simulink model "MIMO_FLOATING_POINT"  (R2023b)
settings: Solver=VariableStepAuto  StartTime=0.0  StopTime=1000  RelTol=1e-3
libraries: dspsigops x80, commchan3 x4, commdigbbndpm3 x2, commfilt2 x2, commsink2 x1, simulink x1, commrandsrc3 x1
(part 2 of 3)

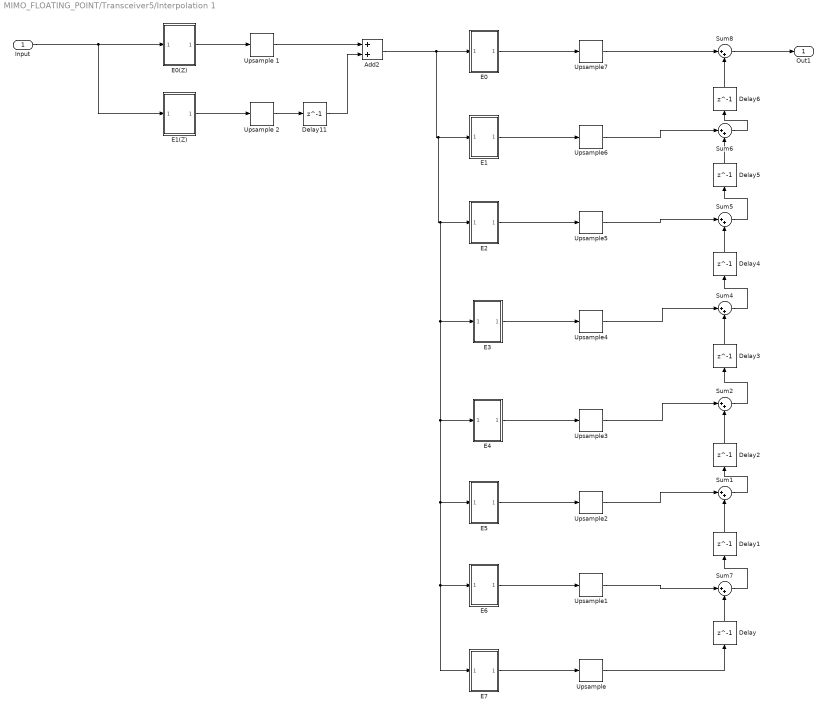
== system MIMO_FLOATING_POINT/Transceiver5/Interpolation 1 ==
  Input : Inport
  Add2 : Sum
  Delay{,1..6,11} (8 alike) : Delay  DelayLength=1
  E0 : Subsystem
  E0(Z) : Subsystem
  E1 : Subsystem
  E1(Z) : Subsystem
  E2 : Subsystem
  E3 : Subsystem
  E4 : Subsystem
  E5 : Subsystem
  E6 : Subsystem
  E7 : Subsystem
  Sum{1..2,4..8} (7 alike) : Sum  Inputs=|++
  Upsample{,1..7} (8 alike) : dspsigops/Upsample  N=8  phase=0  RateOptions=Allow multirate processing  ic=0  mode=Unused parameter value
  Upsample 1 : dspsigops/Upsample  N=2  phase=0  RateOptions=Allow multirate processing  ic=0  mode=Unused parameter value
  Upsample 2 : dspsigops/Upsample  N=2  phase=0  RateOptions=Allow multirate processing  ic=0  mode=Unused parameter value
  Out1 : Outport
  wires:
  Upsample/1 -> Delay/1
  Delay5/1 -> Sum6/2
  Add2/1 -> E7/1(In1), E6/1(In1), E5/1(In1), E4/1(In1), E3/1(In1), E2/1(In1), E1/1(In1), E0/1(In1)
  Upsample6/1 -> Sum6/1
  Delay4/1 -> Sum5/2
  Delay3/1 -> Sum4/2
  E5/1(Out1) -> Upsample2/1
  Sum6/1 -> Delay6/1
  Sum7/1 -> Delay1/1
  E7/1(Out1) -> Upsample/1
  Upsample1/1 -> Sum7/1
  Upsample2/1 -> Sum1/1
  Input/1 -> E1(Z)/1(Input1), E0(Z)/1(Input)
  E0(Z)/1(Out1) -> Upsample 1/1
  Upsample 2/1 -> Delay11/1
  Delay6/1 -> Sum8/2
  E0/1(Out1) -> Upsample7/1
  Delay/1 -> Sum7/2
  E1/1(Out1) -> Upsample6/1
  Delay1/1 -> Sum1/2
  Sum5/1 -> Delay5/1
  Sum4/1 -> Delay4/1
  Upsample5/1 -> Sum5/1
  Upsample 1/1 -> Add2/1
  Sum8/1 -> Out1/1
  Upsample4/1 -> Sum4/1
  Delay11/1 -> Add2/2
  Sum1/1 -> Delay2/1
  Sum2/1 -> Delay3/1
  E6/1(Out1) -> Upsample1/1
  E3/1(Out1) -> Upsample4/1
  Delay2/1 -> Sum2/2
  Upsample7/1 -> Sum8/1
  E1(Z)/1(Output) -> Upsample 2/1
  Upsample3/1 -> Sum2/1
  E2/1(Out1) -> Upsample5/1
  E4/1(Out1) -> Upsample3/1

== system MIMO_FLOATING_POINT/Transceiver5/Subsystem ==
  In1 : Inport
  Delay{,1,4..9} (8 alike) : Delay  DelayLength=1
  Delay2 : Delay  DelayLength=5
  Delay3 : Delay  DelayLength=3
  Gain : Gain
  Gain1 : Gain
  Gain2 : Gain
  Quantizer : Quantizer  QuantizationInterval=1
  Quantizer1 : Quantizer  QuantizationInterval=1
  Quantizer2 : Quantizer  QuantizationInterval=1
  Subtract : Sum  Inputs=+-
  Subtract1 : Sum  Inputs=+-
  Subtract2 : Sum  Inputs=+-
  Sum{,1..2,4,6} (5 alike) : Sum  Inputs=|++
  Sum3 : Sum  Inputs=|+-
  Sum5 : Sum  Inputs=|+-
  Out1 : Outport
  wires:
  Delay/1 -> Sum1/1, Gain/1
  Quantizer/1 -> Subtract/2, Delay2/1
  Sum/1 -> Subtract/1, Quantizer/1
  Sum2/1 -> Subtract2/1, Quantizer2/1
  Delay4/1 -> Gain2/1
  Delay8/1 -> Sum5/2
  Sum4/1 -> Sum5/1, Delay8/1
  Subtract/1 -> Delay/1
  Delay5/1 -> Delay6/1, Sum3/1
  Quantizer1/1 -> Subtract1/2, Delay3/1
  Delay1/1 -> Sum2/1, Gain1/1
  Gain2/1 -> Sum2/2
  Sum1/1 -> Subtract1/1, Quantizer1/1
  Subtract1/1 -> Delay1/1
  Gain1/1 -> Sum1/2
  Sum3/1 -> Delay7/1
  Gain/1 -> Sum/2
  Delay3/1 -> Sum4/1
  Delay7/1 -> Sum4/2
  Subtract2/1 -> Delay4/1
  Quantizer2/1 -> Subtract2/2, Delay5/1
  Delay6/1 -> Sum3/2
  Sum5/1 -> Delay9/1
  Delay2/1 -> Sum6/1
  Delay9/1 -> Sum6/2
  In1/1 -> Sum/1
  Sum6/1 -> Out1/1

== system MIMO_FLOATING_POINT/Transceiver5/Subsystem1 ==
  In1 : Inport
  Delay{,1,4..9} (8 alike) : Delay  DelayLength=1
  Delay2 : Delay  DelayLength=5
  Delay3 : Delay  DelayLength=3
  Gain : Gain
  Gain1 : Gain
  Gain2 : Gain
  Quantizer : Quantizer  QuantizationInterval=1
  Quantizer1 : Quantizer  QuantizationInterval=1
  Quantizer2 : Quantizer  QuantizationInterval=1
  Subtract : Sum  Inputs=+-
  Subtract1 : Sum  Inputs=+-
  Subtract2 : Sum  Inputs=+-
  Sum{,1..2,4,6} (5 alike) : Sum  Inputs=|++
  Sum3 : Sum  Inputs=|+-
  Sum5 : Sum  Inputs=|+-
  Out1 : Outport
  wires:
  Delay/1 -> Sum1/1, Gain/1
  Quantizer/1 -> Subtract/2, Delay2/1
  Sum/1 -> Subtract/1, Quantizer/1
  Sum2/1 -> Subtract2/1, Quantizer2/1
  Delay4/1 -> Gain2/1
  Delay8/1 -> Sum5/2
  Sum4/1 -> Sum5/1, Delay8/1
  Subtract/1 -> Delay/1
  Delay5/1 -> Delay6/1, Sum3/1
  Quantizer1/1 -> Subtract1/2, Delay3/1
  Delay1/1 -> Sum2/1, Gain1/1
  Gain2/1 -> Sum2/2
  Sum1/1 -> Subtract1/1, Quantizer1/1
  Subtract1/1 -> Delay1/1
  Gain1/1 -> Sum1/2
  Sum3/1 -> Delay7/1
  Gain/1 -> Sum/2
  Delay3/1 -> Sum4/1
  Delay7/1 -> Sum4/2
  Subtract2/1 -> Delay4/1
  Quantizer2/1 -> Subtract2/2, Delay5/1
  Delay6/1 -> Sum3/2
  Sum5/1 -> Delay9/1
  Delay2/1 -> Sum6/1
  Delay9/1 -> Sum6/2
  In1/1 -> Sum/1
  Sum6/1 -> Out1/1

== system MIMO_FLOATING_POINT/Transceiver6/ADC 1 ==
  In1 : Inport
  SigmaDelta ADC : Subsystem
  Switch : Switch  Criteria=u2 > Threshold  SaturateOnIntegerOverflow=off  InputSameDT=off
  Zero : Constant  Value=0
  bits 1&0 : Outport
  wires:
  SigmaDelta ADC/1(Out) -> Switch/1, Switch/2
  Zero/1 -> Switch/3
  In1/1 -> SigmaDelta ADC/1(In)
  Switch/1 -> bits 1&0/1

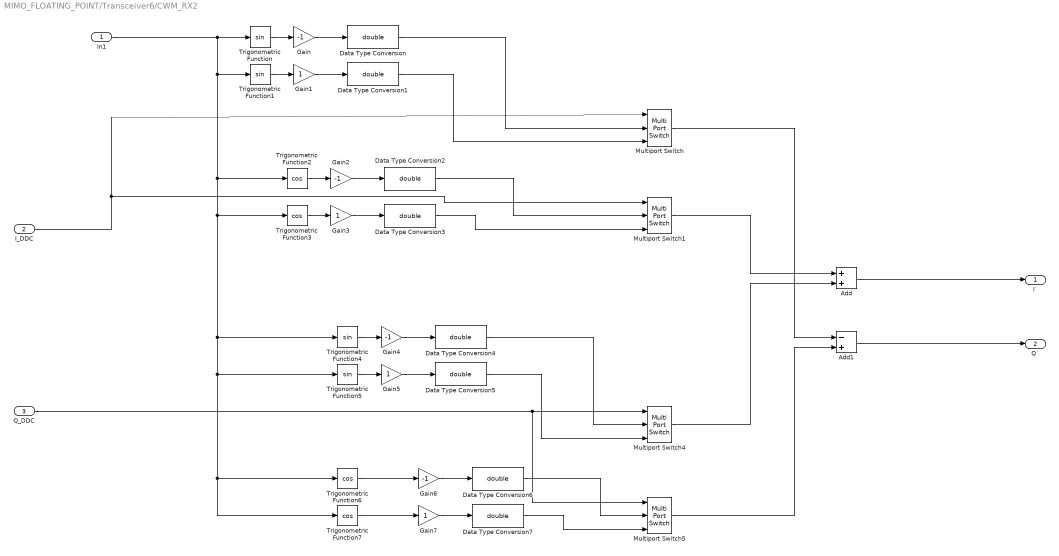
== system MIMO_FLOATING_POINT/Transceiver6/CWM_RX2 ==
  In1 : Inport
  I_DDC : Inport  Port=2
  Q_DDC : Inport  Port=3
  Add : Sum
  Add1 : Sum  Inputs=-+
  Data Type Conversion{,1..7} (8 alike) : DataTypeConversion  OutMin=-1  OutMax=1  OutDataTypeStr=double  RndMeth=Nearest
  Gain{,2,4,6} (4 alike) : Gain  Gain=-1
  Gain{1,3,5,7} (4 alike) : Gain
  Multiport Switch{,1,4..5} (4 alike) : MultiPortSwitch  DataPortOrder=Zero-based contiguous  Inputs=2  zeroidx=on  RndMeth=Nearest  SaturateOnIntegerOverflow=off  InputSameDT=off
  Trigonometric Function{,1,4..5} (4 alike) : Trigonometry
  Trigonometric Function{2..3,6..7} (4 alike) : Trigonometry  Operator=cos
  I` : Outport
  Q` : Outport  Port=2
  wires:
  Multiport Switch/1 -> Add1/1
  Add/1 -> I`/1
  I_DDC/1 -> Multiport Switch1/1, Multiport Switch/1
  Gain2/1 -> Data Type Conversion2/1
  Trigonometric Function5/1 -> Gain5/1
  Data Type Conversion2/1 -> Multiport Switch1/2
  Data Type Conversion1/1 -> Multiport Switch/3
  Gain5/1 -> Data Type Conversion5/1
  Gain4/1 -> Data Type Conversion4/1
  Trigonometric Function1/1 -> Gain1/1
  Data Type Conversion6/1 -> Multiport Switch5/2
  Gain1/1 -> Data Type Conversion1/1
  Gain3/1 -> Data Type Conversion3/1
  Trigonometric Function3/1 -> Gain3/1
  Add1/1 -> Q`/1
  Gain/1 -> Data Type Conversion/1
  Trigonometric Function2/1 -> Gain2/1
  In1/1 -> Trigonometric Function3/1, Trigonometric Function4/1, Trigonometric Function5/1, Trigonometric Function6/1, Trigonometric Function7/1, Trigonometric Function2/1, Trigonometric Function1/1, Trigonometric Function/1
  Q_DDC/1 -> Multiport Switch5/1, Multiport Switch4/1
  Data Type Conversion7/1 -> Multiport Switch5/3
  Data Type Conversion4/1 -> Multiport Switch4/2
  Trigonometric Function6/1 -> Gain6/1
  Gain7/1 -> Data Type Conversion7/1
  Trigonometric Function4/1 -> Gain4/1
  Trigonometric Function/1 -> Gain/1
  Multiport Switch1/1 -> Add/1
  Multiport Switch4/1 -> Add/2
  Trigonometric Function7/1 -> Gain7/1
  Multiport Switch5/1 -> Add1/2
  Data Type Conversion5/1 -> Multiport Switch4/3
  Gain6/1 -> Data Type Conversion6/1
  Data Type Conversion/1 -> Multiport Switch/2
  Data Type Conversion3/1 -> Multiport Switch1/3

== system MIMO_FLOATING_POINT/Transceiver6/CWM_TX_Chain_1 ==
  PHI : Inport
  Processor_I : Inport  Port=2
  Processor_Q : Inport  Port=3
  Add : Sum  OutDataTypeStr=double  RndMeth=Round  SaturateOnIntegerOverflow=on
  Add1 : Sum  OutDataTypeStr=double
  Data Type Conversion{1..4} (4 alike) : DataTypeConversion  Commented=through  OutMin=-1  OutMax=1  OutDataTypeStr=fixdt(1,8,6)  RndMeth=Nearest
  Gain1 : Gain  Gain=-1
  Gain2 : Gain
  Gain3 : Gain
  Gain4 : Gain
  Hamming : Gain  OutDataTypeStr=double
  Hamming1 : Gain  OutDataTypeStr=double
  Product{,1..3} (4 alike) : Product
  Trigonometric Function1 : Trigonometry
  Trigonometric Function2 : Trigonometry  Operator=cos
  Trigonometric Function3 : Trigonometry  Operator=cos
  Trigonometric Function4 : Trigonometry
  I_1 : Outport
  Q_1 : Outport  Port=2
  wires:
  Trigonometric Function2/1 -> Gain2/1
  Gain2/1 -> Data Type Conversion2/1
  Processor_Q/1 -> Product1/2, Product3/2
  Processor_I/1 -> Product2/1, Product/1
  Gain1/1 -> Data Type Conversion1/1
  Product/1 -> Add/1
  Trigonometric Function1/1 -> Gain1/1
  PHI/1 -> Trigonometric Function2/1, Trigonometric Function1/1, Trigonometric Function4/1, Trigonometric Function3/1
  Data Type Conversion1/1 -> Product1/1
  Gain3/1 -> Data Type Conversion3/1
  Product2/1 -> Add1/1
  Data Type Conversion2/1 -> Product/2
  Data Type Conversion4/1 -> Product2/2
  Data Type Conversion3/1 -> Product3/1
  Product3/1 -> Add1/2
  Trigonometric Function3/1 -> Gain3/1
  Product1/1 -> Add/2
  Gain4/1 -> Data Type Conversion4/1
  Trigonometric Function4/1 -> Gain4/1
  Add/1 -> Hamming/1
  Add1/1 -> Hamming1/1
  Hamming/1 -> I_1/1
  Hamming1/1 -> Q_1/1

== system MIMO_FLOATING_POINT/Transceiver6/DDC2 ==
  ODD_I : Inport
  EVEN_Q : Inport  Port=2
  Local_Oscilator1 : DiscretePulseGenerator  PhaseDelay=1  SampleTime=0.02
  Logical Operator : Logic  Operator=NXOR  AllPortsSameDT=off  OutDataTypeStr=boolean
  Logical Operator1 : Logic  Operator=NXOR  AllPortsSameDT=off  OutDataTypeStr=boolean
  NOT : Logic  Operator=NOT  IconShape=distinctive  AllPortsSameDT=off  OutDataTypeStr=boolean
  Scope1 : Scope  NumInputPorts=3
  Scope2 : Scope  NumInputPorts=3
  I_DDC : Outport
  Q_DDC : Outport  Port=2
  wires:
  Logical Operator/1 -> Scope2/3, I_DDC/1
  EVEN_Q/1 -> Scope1/1, Logical Operator1/2
  ODD_I/1 -> Scope2/1, Logical Operator/1
  Logical Operator1/1 -> Scope1/3, Q_DDC/1
  Local_Oscilator1/1 -> NOT/1
  NOT/1 -> Scope1/2, Logical Operator1/1, Scope2/2, Logical Operator/2

== system MIMO_FLOATING_POINT/Transceiver6/DUC2 ==
  I_1 : Inport
  Q_1 : Inport  Port=2
  -cos : Sin  SineType=Sample based  Frequency=2*pi*100  Phase=pi/2  Samples=4  SampleTime=0.01  Offset=3
  -sin1 : Sin  SineType=Sample based  Frequency=(2*pi*100)/4  Samples=4  SampleTime=.01  Offset=2
  Add : Sum
  Constant : Constant  Value=0
  Constant1 : Constant  Value=0
  Gain : Gain  Gain=-1
  Gain1 : Gain  Gain=-1
  Multiport Switch : MultiPortSwitch  DataPortOrder=Specify indices  DataPortIndices={1,0,-1}  RndMeth=Nearest  SaturateOnIntegerOverflow=off  InputSameDT=off
  Multiport Switch1 : MultiPortSwitch  DataPortOrder=Specify indices  DataPortIndices={1,0,-1}  RndMeth=Nearest  SaturateOnIntegerOverflow=off  InputSameDT=off
  Scope : Scope  NumInputPorts=3
  Scope1 : Scope  NumInputPorts=3
  Scope2 : Scope  NumInputPorts=3
  Out2 : Outport
  wires:
  Constant/1 -> Multiport Switch1/3
  Q_1/1 -> Gain1/1, Multiport Switch/2, Scope/1
  I_1/1 -> Gain/1, Scope2/1, Multiport Switch1/2
  Gain1/1 -> Multiport Switch/4
  -sin1/1 -> Scope/2, Multiport Switch/1
  -cos/1 -> Scope2/2, Multiport Switch1/1
  Multiport Switch/1 -> Scope/3, Scope1/2, Add/2
  Add/1 -> Scope1/3, Out2/1
  Multiport Switch1/1 -> Add/1, Scope1/1, Scope2/3
  Constant1/1 -> Multiport Switch/3
  Gain/1 -> Multiport Switch1/4

== system MIMO_FLOATING_POINT/Transceiver6/Inter_Lever2 ==
  bits 1&0 : Inport
  Delay1 : Delay  DelayLength=1  InitialCondition=0
  Delay2 : Delay  DelayLength=1  InitialCondition=0
  Downsample : DownSample  RateOptions=Allow multirate processing
  Downsample1 : DownSample  RateOptions=Allow multirate processing
  Scope1 : Scope  NumInputPorts=3
  ODD_I : Outport
  EVEN_Q : Outport  Port=2
  wires:
  Delay1/1 -> Downsample1/1
  Downsample/1 -> Delay2/1
  Downsample1/1 -> Scope1/3, EVEN_Q/1
  bits 1&0/1 -> Scope1/1, Delay1/1, Downsample/1
  Delay2/1 -> Scope1/2, ODD_I/1

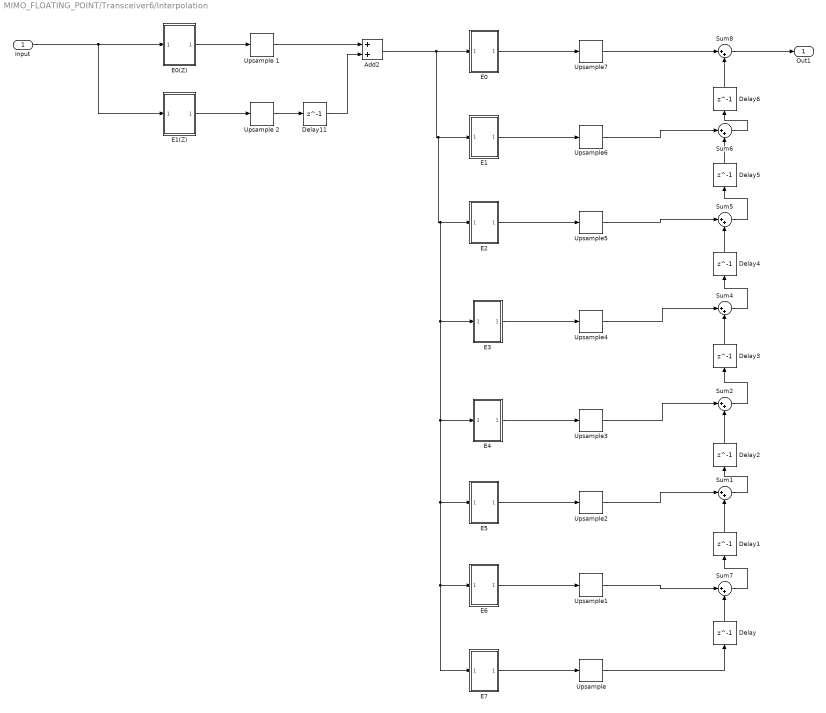
== system MIMO_FLOATING_POINT/Transceiver6/Interpolation  ==
  Input : Inport
  Add2 : Sum
  Delay{,1..6,11} (8 alike) : Delay  DelayLength=1
  E0 : Subsystem
  E0(Z) : Subsystem
  E1 : Subsystem
  E1(Z) : Subsystem
  E2 : Subsystem
  E3 : Subsystem
  E4 : Subsystem
  E5 : Subsystem
  E6 : Subsystem
  E7 : Subsystem
  Sum{1..2,4..8} (7 alike) : Sum  Inputs=|++
  Upsample{,1..7} (8 alike) : dspsigops/Upsample  N=8  phase=0  RateOptions=Allow multirate processing  ic=0  mode=Unused parameter value
  Upsample 1 : dspsigops/Upsample  N=2  phase=0  RateOptions=Allow multirate processing  ic=0  mode=Unused parameter value
  Upsample 2 : dspsigops/Upsample  N=2  phase=0  RateOptions=Allow multirate processing  ic=0  mode=Unused parameter value
  Out1 : Outport
  wires:
  Upsample/1 -> Delay/1
  Delay5/1 -> Sum6/2
  Add2/1 -> E7/1(In1), E6/1(In1), E5/1(In1), E4/1(In1), E3/1(In1), E2/1(In1), E1/1(In1), E0/1(In1)
  Upsample6/1 -> Sum6/1
  Delay4/1 -> Sum5/2
  Delay3/1 -> Sum4/2
  E5/1(Out1) -> Upsample2/1
  Sum6/1 -> Delay6/1
  Sum7/1 -> Delay1/1
  E7/1(Out1) -> Upsample/1
  Upsample1/1 -> Sum7/1
  Upsample2/1 -> Sum1/1
  Input/1 -> E1(Z)/1(Input1), E0(Z)/1(Input)
  E0(Z)/1(Out1) -> Upsample 1/1
  Upsample 2/1 -> Delay11/1
  Delay6/1 -> Sum8/2
  E0/1(Out1) -> Upsample7/1
  Delay/1 -> Sum7/2
  E1/1(Out1) -> Upsample6/1
  Delay1/1 -> Sum1/2
  Sum5/1 -> Delay5/1
  Sum4/1 -> Delay4/1
  Upsample5/1 -> Sum5/1
  Upsample 1/1 -> Add2/1
  Sum8/1 -> Out1/1
  Upsample4/1 -> Sum4/1
  Delay11/1 -> Add2/2
  Sum1/1 -> Delay2/1
  Sum2/1 -> Delay3/1
  E6/1(Out1) -> Upsample1/1
  E3/1(Out1) -> Upsample4/1
  Delay2/1 -> Sum2/2
  Upsample7/1 -> Sum8/1
  E1(Z)/1(Output) -> Upsample 2/1
  Upsample3/1 -> Sum2/1
  E2/1(Out1) -> Upsample5/1
  E4/1(Out1) -> Upsample3/1

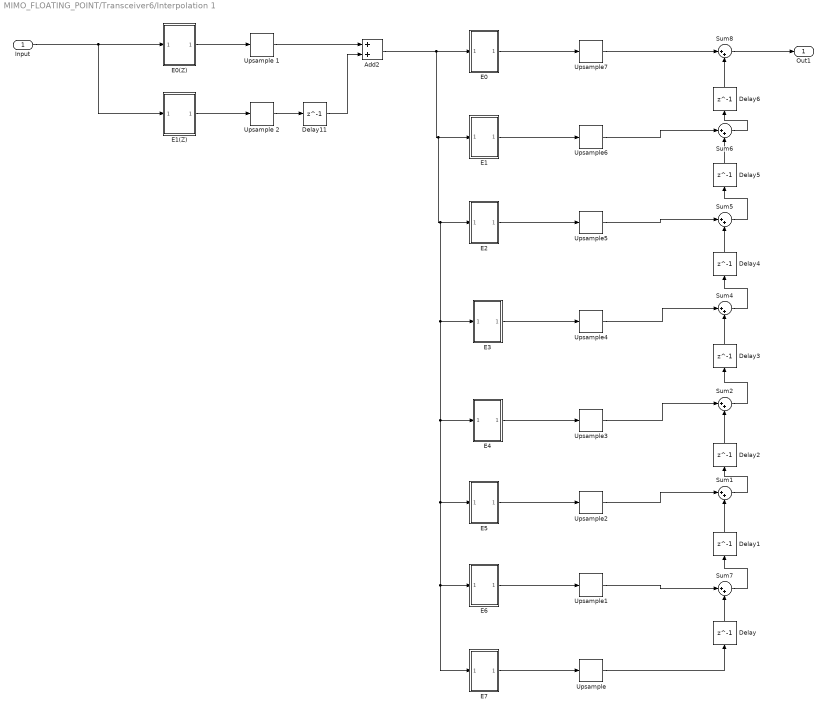
== system MIMO_FLOATING_POINT/Transceiver6/Interpolation 1 ==
  Input : Inport
  Add2 : Sum
  Delay{,1..6,11} (8 alike) : Delay  DelayLength=1
  E0 : Subsystem
  E0(Z) : Subsystem
  E1 : Subsystem
  E1(Z) : Subsystem
  E2 : Subsystem
  E3 : Subsystem
  E4 : Subsystem
  E5 : Subsystem
  E6 : Subsystem
  E7 : Subsystem
  Sum{1..2,4..8} (7 alike) : Sum  Inputs=|++
  Upsample{,1..7} (8 alike) : dspsigops/Upsample  N=8  phase=0  RateOptions=Allow multirate processing  ic=0  mode=Unused parameter value
  Upsample 1 : dspsigops/Upsample  N=2  phase=0  RateOptions=Allow multirate processing  ic=0  mode=Unused parameter value
  Upsample 2 : dspsigops/Upsample  N=2  phase=0  RateOptions=Allow multirate processing  ic=0  mode=Unused parameter value
  Out1 : Outport
  wires:
  Upsample/1 -> Delay/1
  Delay5/1 -> Sum6/2
  Add2/1 -> E7/1(In1), E6/1(In1), E5/1(In1), E4/1(In1), E3/1(In1), E2/1(In1), E1/1(In1), E0/1(In1)
  Upsample6/1 -> Sum6/1
  Delay4/1 -> Sum5/2
  Delay3/1 -> Sum4/2
  E5/1(Out1) -> Upsample2/1
  Sum6/1 -> Delay6/1
  Sum7/1 -> Delay1/1
  E7/1(Out1) -> Upsample/1
  Upsample1/1 -> Sum7/1
  Upsample2/1 -> Sum1/1
  Input/1 -> E1(Z)/1(Input1), E0(Z)/1(Input)
  E0(Z)/1(Out1) -> Upsample 1/1
  Upsample 2/1 -> Delay11/1
  Delay6/1 -> Sum8/2
  E0/1(Out1) -> Upsample7/1
  Delay/1 -> Sum7/2
  E1/1(Out1) -> Upsample6/1
  Delay1/1 -> Sum1/2
  Sum5/1 -> Delay5/1
  Sum4/1 -> Delay4/1
  Upsample5/1 -> Sum5/1
  Upsample 1/1 -> Add2/1
  Sum8/1 -> Out1/1
  Upsample4/1 -> Sum4/1
  Delay11/1 -> Add2/2
  Sum1/1 -> Delay2/1
  Sum2/1 -> Delay3/1
  E6/1(Out1) -> Upsample1/1
  E3/1(Out1) -> Upsample4/1
  Delay2/1 -> Sum2/2
  Upsample7/1 -> Sum8/1
  E1(Z)/1(Output) -> Upsample 2/1
  Upsample3/1 -> Sum2/1
  E2/1(Out1) -> Upsample5/1
  E4/1(Out1) -> Upsample3/1

== system MIMO_FLOATING_POINT/Transceiver6/Subsystem ==
  In1 : Inport
  Delay{,1,4..9} (8 alike) : Delay  DelayLength=1
  Delay2 : Delay  DelayLength=5
  Delay3 : Delay  DelayLength=3
  Gain : Gain
  Gain1 : Gain
  Gain2 : Gain
  Quantizer : Quantizer  QuantizationInterval=1
  Quantizer1 : Quantizer  QuantizationInterval=1
  Quantizer2 : Quantizer  QuantizationInterval=1
  Subtract : Sum  Inputs=+-
  Subtract1 : Sum  Inputs=+-
  Subtract2 : Sum  Inputs=+-
  Sum{,1..2,4,6} (5 alike) : Sum  Inputs=|++
  Sum3 : Sum  Inputs=|+-
  Sum5 : Sum  Inputs=|+-
  Out1 : Outport
  wires:
  Delay/1 -> Sum1/1, Gain/1
  Quantizer/1 -> Subtract/2, Delay2/1
  Sum/1 -> Subtract/1, Quantizer/1
  Sum2/1 -> Subtract2/1, Quantizer2/1
  Delay4/1 -> Gain2/1
  Delay8/1 -> Sum5/2
  Sum4/1 -> Sum5/1, Delay8/1
  Subtract/1 -> Delay/1
  Delay5/1 -> Delay6/1, Sum3/1
  Quantizer1/1 -> Subtract1/2, Delay3/1
  Delay1/1 -> Sum2/1, Gain1/1
  Gain2/1 -> Sum2/2
  Sum1/1 -> Subtract1/1, Quantizer1/1
  Subtract1/1 -> Delay1/1
  Gain1/1 -> Sum1/2
  Sum3/1 -> Delay7/1
  Gain/1 -> Sum/2
  Delay3/1 -> Sum4/1
  Delay7/1 -> Sum4/2
  Subtract2/1 -> Delay4/1
  Quantizer2/1 -> Subtract2/2, Delay5/1
  Delay6/1 -> Sum3/2
  Sum5/1 -> Delay9/1
  Delay2/1 -> Sum6/1
  Delay9/1 -> Sum6/2
  In1/1 -> Sum/1
  Sum6/1 -> Out1/1

== system MIMO_FLOATING_POINT/Transceiver6/Subsystem1 ==
  In1 : Inport
  Delay{,1,4..9} (8 alike) : Delay  DelayLength=1
  Delay2 : Delay  DelayLength=5
  Delay3 : Delay  DelayLength=3
  Gain : Gain
  Gain1 : Gain
  Gain2 : Gain
  Quantizer : Quantizer  QuantizationInterval=1
  Quantizer1 : Quantizer  QuantizationInterval=1
  Quantizer2 : Quantizer  QuantizationInterval=1
  Subtract : Sum  Inputs=+-
  Subtract1 : Sum  Inputs=+-
  Subtract2 : Sum  Inputs=+-
  Sum{,1..2,4,6} (5 alike) : Sum  Inputs=|++
  Sum3 : Sum  Inputs=|+-
  Sum5 : Sum  Inputs=|+-
  Out1 : Outport
  wires:
  Delay/1 -> Sum1/1, Gain/1
  Quantizer/1 -> Subtract/2, Delay2/1
  Sum/1 -> Subtract/1, Quantizer/1
  Sum2/1 -> Subtract2/1, Quantizer2/1
  Delay4/1 -> Gain2/1
  Delay8/1 -> Sum5/2
  Sum4/1 -> Sum5/1, Delay8/1
  Subtract/1 -> Delay/1
  Delay5/1 -> Delay6/1, Sum3/1
  Quantizer1/1 -> Subtract1/2, Delay3/1
  Delay1/1 -> Sum2/1, Gain1/1
  Gain2/1 -> Sum2/2
  Sum1/1 -> Subtract1/1, Quantizer1/1
  Subtract1/1 -> Delay1/1
  Gain1/1 -> Sum1/2
  Sum3/1 -> Delay7/1
  Gain/1 -> Sum/2
  Delay3/1 -> Sum4/1
  Delay7/1 -> Sum4/2
  Subtract2/1 -> Delay4/1
  Quantizer2/1 -> Subtract2/2, Delay5/1
  Delay6/1 -> Sum3/2
  Sum5/1 -> Delay9/1
  Delay2/1 -> Sum6/1
  Delay9/1 -> Sum6/2
  In1/1 -> Sum/1
  Sum6/1 -> Out1/1

== system MIMO_FLOATING_POINT/Transceiver7/ADC 1 ==
  In1 : Inport
  SigmaDelta ADC : Subsystem
  Switch : Switch  Criteria=u2 > Threshold  SaturateOnIntegerOverflow=off  InputSameDT=off
  Zero : Constant  Value=0
  bits 1&0 : Outport
  wires:
  SigmaDelta ADC/1(Out) -> Switch/1, Switch/2
  Zero/1 -> Switch/3
  In1/1 -> SigmaDelta ADC/1(In)
  Switch/1 -> bits 1&0/1

== system MIMO_FLOATING_POINT/Transceiver7/CWM_RX2 ==
  In1 : Inport
  I_DDC : Inport  Port=2
  Q_DDC : Inport  Port=3
  Add : Sum
  Add1 : Sum  Inputs=-+
  Data Type Conversion{,1..7} (8 alike) : DataTypeConversion  OutMin=-1  OutMax=1  OutDataTypeStr=double  RndMeth=Nearest
  Gain{,2,4,6} (4 alike) : Gain  Gain=-1
  Gain{1,3,5,7} (4 alike) : Gain
  Multiport Switch{,1,4..5} (4 alike) : MultiPortSwitch  DataPortOrder=Zero-based contiguous  Inputs=2  zeroidx=on  RndMeth=Nearest  SaturateOnIntegerOverflow=off  InputSameDT=off
  Trigonometric Function{,1,4..5} (4 alike) : Trigonometry
  Trigonometric Function{2..3,6..7} (4 alike) : Trigonometry  Operator=cos
  I` : Outport
  Q` : Outport  Port=2
  wires:
  Multiport Switch/1 -> Add1/1
  Add/1 -> I`/1
  I_DDC/1 -> Multiport Switch1/1, Multiport Switch/1
  Gain2/1 -> Data Type Conversion2/1
  Trigonometric Function5/1 -> Gain5/1
  Data Type Conversion2/1 -> Multiport Switch1/2
  Data Type Conversion1/1 -> Multiport Switch/3
  Gain5/1 -> Data Type Conversion5/1
  Gain4/1 -> Data Type Conversion4/1
  Trigonometric Function1/1 -> Gain1/1
  Data Type Conversion6/1 -> Multiport Switch5/2
  Gain1/1 -> Data Type Conversion1/1
  Gain3/1 -> Data Type Conversion3/1
  Trigonometric Function3/1 -> Gain3/1
  Add1/1 -> Q`/1
  Gain/1 -> Data Type Conversion/1
  Trigonometric Function2/1 -> Gain2/1
  In1/1 -> Trigonometric Function3/1, Trigonometric Function4/1, Trigonometric Function5/1, Trigonometric Function6/1, Trigonometric Function7/1, Trigonometric Function2/1, Trigonometric Function1/1, Trigonometric Function/1
  Q_DDC/1 -> Multiport Switch5/1, Multiport Switch4/1
  Data Type Conversion7/1 -> Multiport Switch5/3
  Data Type Conversion4/1 -> Multiport Switch4/2
  Trigonometric Function6/1 -> Gain6/1
  Gain7/1 -> Data Type Conversion7/1
  Trigonometric Function4/1 -> Gain4/1
  Trigonometric Function/1 -> Gain/1
  Multiport Switch1/1 -> Add/1
  Multiport Switch4/1 -> Add/2
  Trigonometric Function7/1 -> Gain7/1
  Multiport Switch5/1 -> Add1/2
  Data Type Conversion5/1 -> Multiport Switch4/3
  Gain6/1 -> Data Type Conversion6/1
  Data Type Conversion/1 -> Multiport Switch/2
  Data Type Conversion3/1 -> Multiport Switch1/3

== system MIMO_FLOATING_POINT/Transceiver7/CWM_TX_Chain_1 ==
  PHI : Inport
  Processor_I : Inport  Port=2
  Processor_Q : Inport  Port=3
  Add : Sum  OutDataTypeStr=double  RndMeth=Round  SaturateOnIntegerOverflow=on
  Add1 : Sum  OutDataTypeStr=double
  Data Type Conversion{1..4} (4 alike) : DataTypeConversion  Commented=through  OutMin=-1  OutMax=1  OutDataTypeStr=fixdt(1,8,6)  RndMeth=Nearest
  Gain1 : Gain  Gain=-1
  Gain2 : Gain
  Gain3 : Gain
  Gain4 : Gain
  Hamming : Gain  OutDataTypeStr=double
  Hamming1 : Gain  OutDataTypeStr=double
  Product{,1..3} (4 alike) : Product
  Trigonometric Function1 : Trigonometry
  Trigonometric Function2 : Trigonometry  Operator=cos
  Trigonometric Function3 : Trigonometry  Operator=cos
  Trigonometric Function4 : Trigonometry
  I_1 : Outport
  Q_1 : Outport  Port=2
  wires:
  Trigonometric Function2/1 -> Gain2/1
  Gain2/1 -> Data Type Conversion2/1
  Processor_Q/1 -> Product1/2, Product3/2
  Processor_I/1 -> Product2/1, Product/1
  Gain1/1 -> Data Type Conversion1/1
  Product/1 -> Add/1
  Trigonometric Function1/1 -> Gain1/1
  PHI/1 -> Trigonometric Function2/1, Trigonometric Function1/1, Trigonometric Function4/1, Trigonometric Function3/1
  Data Type Conversion1/1 -> Product1/1
  Gain3/1 -> Data Type Conversion3/1
  Product2/1 -> Add1/1
  Data Type Conversion2/1 -> Product/2
  Data Type Conversion4/1 -> Product2/2
  Data Type Conversion3/1 -> Product3/1
  Product3/1 -> Add1/2
  Trigonometric Function3/1 -> Gain3/1
  Product1/1 -> Add/2
  Gain4/1 -> Data Type Conversion4/1
  Trigonometric Function4/1 -> Gain4/1
  Add/1 -> Hamming/1
  Add1/1 -> Hamming1/1
  Hamming/1 -> I_1/1
  Hamming1/1 -> Q_1/1

== system MIMO_FLOATING_POINT/Transceiver7/DDC2 ==
  ODD_I : Inport
  EVEN_Q : Inport  Port=2
  Local_Oscilator1 : DiscretePulseGenerator  PhaseDelay=1  SampleTime=0.02
  Logical Operator : Logic  Operator=NXOR  AllPortsSameDT=off  OutDataTypeStr=boolean
  Logical Operator1 : Logic  Operator=NXOR  AllPortsSameDT=off  OutDataTypeStr=boolean
  NOT : Logic  Operator=NOT  IconShape=distinctive  AllPortsSameDT=off  OutDataTypeStr=boolean
  Scope1 : Scope  NumInputPorts=3
  Scope2 : Scope  NumInputPorts=3
  I_DDC : Outport
  Q_DDC : Outport  Port=2
  wires:
  Logical Operator/1 -> Scope2/3, I_DDC/1
  EVEN_Q/1 -> Scope1/1, Logical Operator1/2
  ODD_I/1 -> Scope2/1, Logical Operator/1
  Logical Operator1/1 -> Scope1/3, Q_DDC/1
  Local_Oscilator1/1 -> NOT/1
  NOT/1 -> Scope1/2, Logical Operator1/1, Scope2/2, Logical Operator/2

== system MIMO_FLOATING_POINT/Transceiver7/DUC2 ==
  I_1 : Inport
  Q_1 : Inport  Port=2
  -cos : Sin  SineType=Sample based  Frequency=2*pi*100  Phase=pi/2  Samples=4  SampleTime=0.01  Offset=3
  -sin1 : Sin  SineType=Sample based  Frequency=(2*pi*100)/4  Samples=4  SampleTime=.01  Offset=2
  Add : Sum
  Constant : Constant  Value=0
  Constant1 : Constant  Value=0
  Gain : Gain  Gain=-1
  Gain1 : Gain  Gain=-1
  Multiport Switch : MultiPortSwitch  DataPortOrder=Specify indices  DataPortIndices={1,0,-1}  RndMeth=Nearest  SaturateOnIntegerOverflow=off  InputSameDT=off
  Multiport Switch1 : MultiPortSwitch  DataPortOrder=Specify indices  DataPortIndices={1,0,-1}  RndMeth=Nearest  SaturateOnIntegerOverflow=off  InputSameDT=off
  Scope : Scope  NumInputPorts=3
  Scope1 : Scope  NumInputPorts=3
  Scope2 : Scope  NumInputPorts=3
  Out2 : Outport
  wires:
  Constant/1 -> Multiport Switch1/3
  Q_1/1 -> Gain1/1, Multiport Switch/2, Scope/1
  I_1/1 -> Gain/1, Scope2/1, Multiport Switch1/2
  Gain1/1 -> Multiport Switch/4
  -sin1/1 -> Scope/2, Multiport Switch/1
  -cos/1 -> Scope2/2, Multiport Switch1/1
  Multiport Switch/1 -> Scope/3, Scope1/2, Add/2
  Add/1 -> Scope1/3, Out2/1
  Multiport Switch1/1 -> Add/1, Scope1/1, Scope2/3
  Constant1/1 -> Multiport Switch/3
  Gain/1 -> Multiport Switch1/4

== system MIMO_FLOATING_POINT/Transceiver7/Inter_Lever2 ==
  bits 1&0 : Inport
  Delay1 : Delay  DelayLength=1  InitialCondition=0
  Delay2 : Delay  DelayLength=1  InitialCondition=0
  Downsample : DownSample  RateOptions=Allow multirate processing
  Downsample1 : DownSample  RateOptions=Allow multirate processing
  Scope1 : Scope  NumInputPorts=3
  ODD_I : Outport
  EVEN_Q : Outport  Port=2
  wires:
  Delay1/1 -> Downsample1/1
  Downsample/1 -> Delay2/1
  Downsample1/1 -> Scope1/3, EVEN_Q/1
  bits 1&0/1 -> Scope1/1, Delay1/1, Downsample/1
  Delay2/1 -> Scope1/2, ODD_I/1

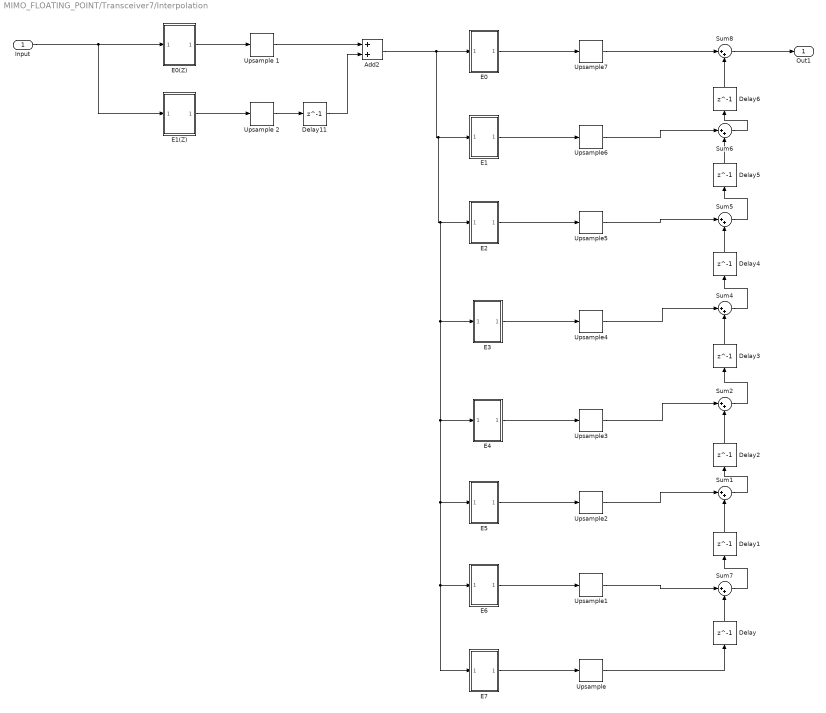
== system MIMO_FLOATING_POINT/Transceiver7/Interpolation  ==
  Input : Inport
  Add2 : Sum
  Delay{,1..6,11} (8 alike) : Delay  DelayLength=1
  E0 : Subsystem
  E0(Z) : Subsystem
  E1 : Subsystem
  E1(Z) : Subsystem
  E2 : Subsystem
  E3 : Subsystem
  E4 : Subsystem
  E5 : Subsystem
  E6 : Subsystem
  E7 : Subsystem
  Sum{1..2,4..8} (7 alike) : Sum  Inputs=|++
  Upsample{,1..7} (8 alike) : dspsigops/Upsample  N=8  phase=0  RateOptions=Allow multirate processing  ic=0  mode=Unused parameter value
  Upsample 1 : dspsigops/Upsample  N=2  phase=0  RateOptions=Allow multirate processing  ic=0  mode=Unused parameter value
  Upsample 2 : dspsigops/Upsample  N=2  phase=0  RateOptions=Allow multirate processing  ic=0  mode=Unused parameter value
  Out1 : Outport
  wires:
  Upsample/1 -> Delay/1
  Delay5/1 -> Sum6/2
  Add2/1 -> E7/1(In1), E6/1(In1), E5/1(In1), E4/1(In1), E3/1(In1), E2/1(In1), E1/1(In1), E0/1(In1)
  Upsample6/1 -> Sum6/1
  Delay4/1 -> Sum5/2
  Delay3/1 -> Sum4/2
  E5/1(Out1) -> Upsample2/1
  Sum6/1 -> Delay6/1
  Sum7/1 -> Delay1/1
  E7/1(Out1) -> Upsample/1
  Upsample1/1 -> Sum7/1
  Upsample2/1 -> Sum1/1
  Input/1 -> E1(Z)/1(Input1), E0(Z)/1(Input)
  E0(Z)/1(Out1) -> Upsample 1/1
  Upsample 2/1 -> Delay11/1
  Delay6/1 -> Sum8/2
  E0/1(Out1) -> Upsample7/1
  Delay/1 -> Sum7/2
  E1/1(Out1) -> Upsample6/1
  Delay1/1 -> Sum1/2
  Sum5/1 -> Delay5/1
  Sum4/1 -> Delay4/1
  Upsample5/1 -> Sum5/1
  Upsample 1/1 -> Add2/1
  Sum8/1 -> Out1/1
  Upsample4/1 -> Sum4/1
  Delay11/1 -> Add2/2
  Sum1/1 -> Delay2/1
  Sum2/1 -> Delay3/1
  E6/1(Out1) -> Upsample1/1
  E3/1(Out1) -> Upsample4/1
  Delay2/1 -> Sum2/2
  Upsample7/1 -> Sum8/1
  E1(Z)/1(Output) -> Upsample 2/1
  Upsample3/1 -> Sum2/1
  E2/1(Out1) -> Upsample5/1
  E4/1(Out1) -> Upsample3/1

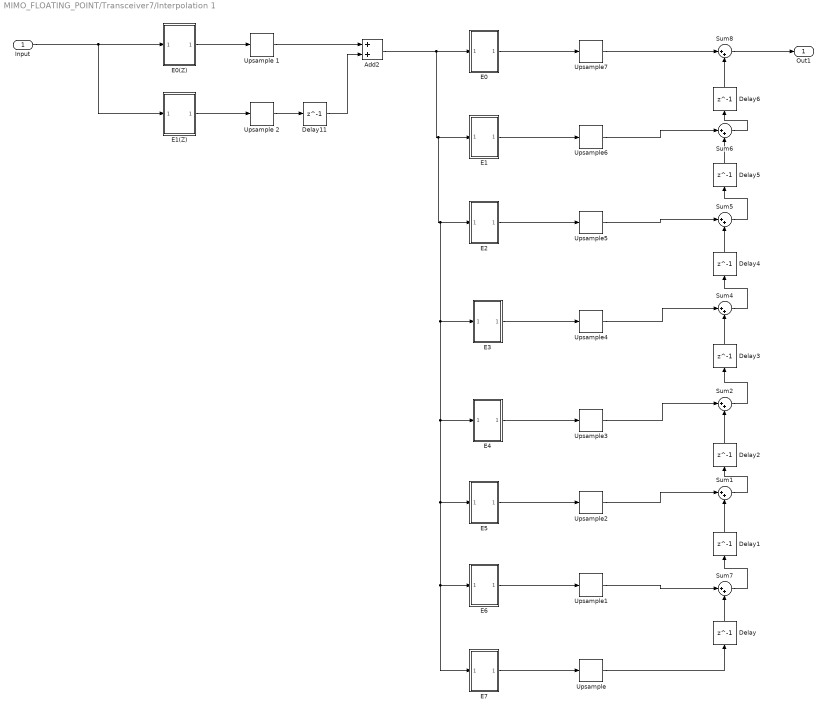
== system MIMO_FLOATING_POINT/Transceiver7/Interpolation 1 ==
  Input : Inport
  Add2 : Sum
  Delay{,1..6,11} (8 alike) : Delay  DelayLength=1
  E0 : Subsystem
  E0(Z) : Subsystem
  E1 : Subsystem
  E1(Z) : Subsystem
  E2 : Subsystem
  E3 : Subsystem
  E4 : Subsystem
  E5 : Subsystem
  E6 : Subsystem
  E7 : Subsystem
  Sum{1..2,4..8} (7 alike) : Sum  Inputs=|++
  Upsample{,1..7} (8 alike) : dspsigops/Upsample  N=8  phase=0  RateOptions=Allow multirate processing  ic=0  mode=Unused parameter value
  Upsample 1 : dspsigops/Upsample  N=2  phase=0  RateOptions=Allow multirate processing  ic=0  mode=Unused parameter value
  Upsample 2 : dspsigops/Upsample  N=2  phase=0  RateOptions=Allow multirate processing  ic=0  mode=Unused parameter value
  Out1 : Outport
  wires:
  Upsample/1 -> Delay/1
  Delay5/1 -> Sum6/2
  Add2/1 -> E7/1(In1), E6/1(In1), E5/1(In1), E4/1(In1), E3/1(In1), E2/1(In1), E1/1(In1), E0/1(In1)
  Upsample6/1 -> Sum6/1
  Delay4/1 -> Sum5/2
  Delay3/1 -> Sum4/2
  E5/1(Out1) -> Upsample2/1
  Sum6/1 -> Delay6/1
  Sum7/1 -> Delay1/1
  E7/1(Out1) -> Upsample/1
  Upsample1/1 -> Sum7/1
  Upsample2/1 -> Sum1/1
  Input/1 -> E1(Z)/1(Input1), E0(Z)/1(Input)
  E0(Z)/1(Out1) -> Upsample 1/1
  Upsample 2/1 -> Delay11/1
  Delay6/1 -> Sum8/2
  E0/1(Out1) -> Upsample7/1
  Delay/1 -> Sum7/2
  E1/1(Out1) -> Upsample6/1
  Delay1/1 -> Sum1/2
  Sum5/1 -> Delay5/1
  Sum4/1 -> Delay4/1
  Upsample5/1 -> Sum5/1
  Upsample 1/1 -> Add2/1
  Sum8/1 -> Out1/1
  Upsample4/1 -> Sum4/1
  Delay11/1 -> Add2/2
  Sum1/1 -> Delay2/1
  Sum2/1 -> Delay3/1
  E6/1(Out1) -> Upsample1/1
  E3/1(Out1) -> Upsample4/1
  Delay2/1 -> Sum2/2
  Upsample7/1 -> Sum8/1
  E1(Z)/1(Output) -> Upsample 2/1
  Upsample3/1 -> Sum2/1
  E2/1(Out1) -> Upsample5/1
  E4/1(Out1) -> Upsample3/1

== system MIMO_FLOATING_POINT/Transceiver7/Subsystem ==
  In1 : Inport
  Delay{,1,4..9} (8 alike) : Delay  DelayLength=1
  Delay2 : Delay  DelayLength=5
  Delay3 : Delay  DelayLength=3
  Gain : Gain
  Gain1 : Gain
  Gain2 : Gain
  Quantizer : Quantizer  QuantizationInterval=1
  Quantizer1 : Quantizer  QuantizationInterval=1
  Quantizer2 : Quantizer  QuantizationInterval=1
  Subtract : Sum  Inputs=+-
  Subtract1 : Sum  Inputs=+-
  Subtract2 : Sum  Inputs=+-
  Sum{,1..2,4,6} (5 alike) : Sum  Inputs=|++
  Sum3 : Sum  Inputs=|+-
  Sum5 : Sum  Inputs=|+-
  Out1 : Outport
  wires:
  Delay/1 -> Sum1/1, Gain/1
  Quantizer/1 -> Subtract/2, Delay2/1
  Sum/1 -> Subtract/1, Quantizer/1
  Sum2/1 -> Subtract2/1, Quantizer2/1
  Delay4/1 -> Gain2/1
  Delay8/1 -> Sum5/2
  Sum4/1 -> Sum5/1, Delay8/1
  Subtract/1 -> Delay/1
  Delay5/1 -> Delay6/1, Sum3/1
  Quantizer1/1 -> Subtract1/2, Delay3/1
  Delay1/1 -> Sum2/1, Gain1/1
  Gain2/1 -> Sum2/2
  Sum1/1 -> Subtract1/1, Quantizer1/1
  Subtract1/1 -> Delay1/1
  Gain1/1 -> Sum1/2
  Sum3/1 -> Delay7/1
  Gain/1 -> Sum/2
  Delay3/1 -> Sum4/1
  Delay7/1 -> Sum4/2
  Subtract2/1 -> Delay4/1
  Quantizer2/1 -> Subtract2/2, Delay5/1
  Delay6/1 -> Sum3/2
  Sum5/1 -> Delay9/1
  Delay2/1 -> Sum6/1
  Delay9/1 -> Sum6/2
  In1/1 -> Sum/1
  Sum6/1 -> Out1/1

== system MIMO_FLOATING_POINT/Transceiver7/Subsystem1 ==
  In1 : Inport
  Delay{,1,4..9} (8 alike) : Delay  DelayLength=1
  Delay2 : Delay  DelayLength=5
  Delay3 : Delay  DelayLength=3
  Gain : Gain
  Gain1 : Gain
  Gain2 : Gain
  Quantizer : Quantizer  QuantizationInterval=1
  Quantizer1 : Quantizer  QuantizationInterval=1
  Quantizer2 : Quantizer  QuantizationInterval=1
  Subtract : Sum  Inputs=+-
  Subtract1 : Sum  Inputs=+-
  Subtract2 : Sum  Inputs=+-
  Sum{,1..2,4,6} (5 alike) : Sum  Inputs=|++
  Sum3 : Sum  Inputs=|+-
  Sum5 : Sum  Inputs=|+-
  Out1 : Outport
  wires:
  Delay/1 -> Sum1/1, Gain/1
  Quantizer/1 -> Subtract/2, Delay2/1
  Sum/1 -> Subtract/1, Quantizer/1
  Sum2/1 -> Subtract2/1, Quantizer2/1
  Delay4/1 -> Gain2/1
  Delay8/1 -> Sum5/2
  Sum4/1 -> Sum5/1, Delay8/1
  Subtract/1 -> Delay/1
  Delay5/1 -> Delay6/1, Sum3/1
  Quantizer1/1 -> Subtract1/2, Delay3/1
  Delay1/1 -> Sum2/1, Gain1/1
  Gain2/1 -> Sum2/2
  Sum1/1 -> Subtract1/1, Quantizer1/1
  Subtract1/1 -> Delay1/1
  Gain1/1 -> Sum1/2
  Sum3/1 -> Delay7/1
  Gain/1 -> Sum/2
  Delay3/1 -> Sum4/1
  Delay7/1 -> Sum4/2
  Subtract2/1 -> Delay4/1
  Quantizer2/1 -> Subtract2/2, Delay5/1
  Delay6/1 -> Sum3/2
  Sum5/1 -> Delay9/1
  Delay2/1 -> Sum6/1
  Delay9/1 -> Sum6/2
  In1/1 -> Sum/1
  Sum6/1 -> Out1/1

== system MIMO_FLOATING_POINT/Transceiver/ADC 1/SigmaDelta ADC ==
  note: c1
  In : Inport
  Discrete Transfer Fcn : DiscreteTransferFcn  Denominator=[1 -1]
  Discrete Transfer Fcn1 : DiscreteTransferFcn  Numerator=[1 0]  Denominator=[1 -1]
  Discrete Transfer Fcn2 : DiscreteTransferFcn  Denominator=[1 -1]
  Discrete Transfer Fcn3 : DiscreteTransferFcn  Numerator=[1 0]  Denominator=[1 -1]
  Discrete Transfer Fcn4 : DiscreteTransferFcn  Denominator=[1 -1]
  Discrete Transfer Fcn5 : DiscreteTransferFcn  Numerator=[1 0]  Denominator=[1 -1]
  Sign : Signum
  Sum : Sum  Inputs=-++  InputSameDT=on  SaturateOnIntegerOverflow=on  OutDataTypeStr=Inherit: Same as first input
  Sum1 : Sum  Inputs=-+  InputSameDT=on  SaturateOnIntegerOverflow=on  OutDataTypeStr=Inherit: Same as first input
  Sum3 : Sum  Inputs=-+  InputSameDT=on  SaturateOnIntegerOverflow=on  OutDataTypeStr=Inherit: Same as first input
  Sum4 : Sum  Inputs=++++++  InputSameDT=on  SaturateOnIntegerOverflow=on  OutDataTypeStr=Inherit: Same as first input
  a : Gain  Gain=-1  SaturateOnIntegerOverflow=on  OutDataTypeStr=Inherit: Same as input  ParamDataTypeStr=Inherit: Same as input
  a1 : Gain  Gain=0.556869897897495  SaturateOnIntegerOverflow=on  OutDataTypeStr=Inherit: Same as input  ParamDataTypeStr=Inherit: Same as input
  a2 : Gain  Gain=-0.556869897925717  SaturateOnIntegerOverflow=on  OutDataTypeStr=Inherit: Same as input  ParamDataTypeStr=Inherit: Same as input
  a3 : Gain  Gain=5.57074843011795e-10  SaturateOnIntegerOverflow=on  OutDataTypeStr=Inherit: Same as input  ParamDataTypeStr=Inherit: Same as input
  a4 : Gain  Gain=-0.239860502762260  SaturateOnIntegerOverflow=on  OutDataTypeStr=Inherit: Same as input  ParamDataTypeStr=Inherit: Same as input
  a5 : Gain  Gain=-0.0411685762497780  SaturateOnIntegerOverflow=on  OutDataTypeStr=Inherit: Same as input  ParamDataTypeStr=Inherit: Same as input
  a6 : Gain  Gain=0.0229325751731016  SaturateOnIntegerOverflow=on  OutDataTypeStr=Inherit: Same as input  ParamDataTypeStr=Inherit: Same as input
  gc1 : Gain  Gain=2.00000000000000  SaturateOnIntegerOverflow=on  OutDataTypeStr=Inherit: Same as input  ParamDataTypeStr=Inherit: Same as input
  gc2 : Gain  Gain=2.07602752770857  SaturateOnIntegerOverflow=on  OutDataTypeStr=Inherit: Same as input  ParamDataTypeStr=Inherit: Same as input
  gc3 : Gain  Gain=1.92397247229143  SaturateOnIntegerOverflow=on  OutDataTypeStr=Inherit: Same as input  ParamDataTypeStr=Inherit: Same as input
  Out : Outport
  wires:
  gc1/1 -> Sum/1
  a5/1 -> Sum4/2
  Discrete Transfer Fcn2/1 -> Discrete Transfer Fcn3/1, a3/1
  Sum4/1 -> Sign/1
  Sum1/1 -> Discrete Transfer Fcn2/1
  Sum/1 -> Discrete Transfer Fcn/1
  a1/1 -> Sum4/6
  gc2/1 -> Sum1/1
  a/1 -> Sum/3
  Discrete Transfer Fcn3/1 -> a4/1, Sum3/2, gc2/1
  Discrete Transfer Fcn5/1 -> a6/1, gc3/1
  Discrete Transfer Fcn1/1 -> a2/1, gc1/1, Sum1/2
  In/1 -> Sum/2
  Sign/1 -> Out/1, a/1
  gc3/1 -> Sum3/1
  a3/1 -> Sum4/4
  a4/1 -> Sum4/3
  a2/1 -> Sum4/5
  Discrete Transfer Fcn/1 -> Discrete Transfer Fcn1/1, a1/1
  Sum3/1 -> Discrete Transfer Fcn4/1
  Discrete Transfer Fcn4/1 -> Discrete Transfer Fcn5/1, a5/1
  a6/1 -> Sum4/1

== system MIMO_FLOATING_POINT/Transceiver/Interpolation /E0 ==
  In1 : Inport
  Delay3 : Delay  DelayLength=1
  Delay4 : Delay  DelayLength=1
  Delay5 : Delay  DelayLength=1
  Gain : Gain  Gain=35
  Gain1 : Gain  Gain=315
  Gain2 : Gain  Gain=161
  Gain3 : Gain
  Sum : Sum
  Sum1 : Sum
  Sum2 : Sum
  Out1 : Outport
  wires:
  In1/1 -> Gain2/1, Gain3/1, Gain1/1, Gain/1
  Sum1/1 -> Delay5/1
  Sum/1 -> Delay4/1
  Gain1/1 -> Sum/1
  Delay3/1 -> Sum/2
  Delay4/1 -> Sum1/2
  Gain3/1 -> Sum2/1
  Delay5/1 -> Sum2/2
  Gain/1 -> Delay3/1
  Sum2/1 -> Out1/1
  Gain2/1 -> Sum1/1

== system MIMO_FLOATING_POINT/Transceiver/Interpolation /E0(Z) ==
  Input : Inport
  Delay : Delay  DelayLength=5
  Gain : Gain  Gain=0.5
  Out1 : Outport
  wires:
  Input/1 -> Gain/1
  Delay/1 -> Out1/1
  Gain/1 -> Delay/1

== system MIMO_FLOATING_POINT/Transceiver/Interpolation /E1 ==
  In1 : Inport
  Delay3 : Delay  DelayLength=1
  Delay4 : Delay  DelayLength=1
  Delay5 : Delay  DelayLength=1
  Gain : Gain  Gain=20
  Gain1 : Gain  Gain=284
  Gain2 : Gain  Gain=204
  Gain3 : Gain  Gain=4
  Sum : Sum
  Sum1 : Sum
  Sum2 : Sum
  Out1 : Outport
  wires:
  In1/1 -> Gain2/1, Gain3/1, Gain1/1, Gain/1
  Sum1/1 -> Delay5/1
  Sum/1 -> Delay4/1
  Gain1/1 -> Sum/1
  Delay3/1 -> Sum/2
  Delay4/1 -> Sum1/2
  Gain3/1 -> Sum2/1
  Delay5/1 -> Sum2/2
  Gain/1 -> Delay3/1
  Sum2/1 -> Out1/1
  Gain2/1 -> Sum1/1

== system MIMO_FLOATING_POINT/Transceiver/Interpolation /E1(Z) ==
  Input1 : Inport
  10-12 : Gain  Gain=0.3078
  2-20 : Gain  Gain=0.0011
  4-18 : Gain  Gain=-0.0072
  6-16 : Gain  Gain=0.0263
  8-14 : Gain  Gain=-0.078
  Add{7..10,12..16} (9 alike) : Sum
  Delay{21,23,25,27,29,31,33,35,37} (9 alike) : Delay  DelayLength=1
  Output : Outport
  wires:
  8-14/1 -> Add13/1, Add9/1
  Delay29/1 -> Add12/2  "x[n-11]"
  Add14/1 -> Delay35/1
  Input1/1 -> 2-20/1, 4-18/1, 6-16/1, 8-14/1, 10-12/1
  Add8/1 -> Delay25/1
  4-18/1 -> Add15/1, Add7/1
  Delay33/1 -> Add14/2  "x[n-15]"
  Add12/1 -> Delay31/1
  10-12/1 -> Add10/1, Add12/1
  Add9/1 -> Delay27/1
  Add16/1 -> Output/1
  Delay37/1 -> Add16/2  "x[n-19]"
  6-16/1 -> Add14/1, Add8/1
  Delay25/1 -> Add9/2  "x[n-7]"
  Add7/1 -> Delay23/1
  Add15/1 -> Delay37/1
  Delay23/1 -> Add8/2  "x[n-5]"
  Delay27/1 -> Add10/2  "x[n-9]"
  Delay31/1 -> Add13/2  "x[n-13]"
  Delay35/1 -> Add15/2  "x[n-17]"
  Delay21/1 -> Add7/2  "x[n-3]"
  2-20/1 -> Delay21/1, Add16/1
  Add13/1 -> Delay33/1
  Add10/1 -> Delay29/1

== system MIMO_FLOATING_POINT/Transceiver/Interpolation /E2 ==
  In1 : Inport
  Delay3 : Delay  DelayLength=1
  Delay4 : Delay  DelayLength=1
  Delay5 : Delay  DelayLength=1
  Gain : Gain  Gain=10
  Gain1 : Gain  Gain=246
  Sum : Sum
  Sum1 : Sum
  Sum2 : Sum
  Out1 : Outport
  wires:
  In1/1 -> Gain1/1, Gain/1
  Sum1/1 -> Delay5/1
  Sum/1 -> Delay4/1
  Gain1/1 -> Sum1/1, Sum/1
  Delay3/1 -> Sum/2
  Delay4/1 -> Sum1/2
  Gain/1 -> Sum2/1, Delay3/1
  Delay5/1 -> Sum2/2
  Sum2/1 -> Out1/1

== system MIMO_FLOATING_POINT/Transceiver/Interpolation /E3 ==
  In1 : Inport
  Delay3 : Delay  DelayLength=1
  Delay4 : Delay  DelayLength=1
  Delay5 : Delay  DelayLength=1
  Gain : Gain  Gain=4
  Gain1 : Gain  Gain=204
  Gain2 : Gain  Gain=284
  Gain3 : Gain  Gain=20
  Sum : Sum
  Sum1 : Sum
  Sum2 : Sum
  Out1 : Outport
  wires:
  In1/1 -> Gain2/1, Gain3/1, Gain1/1, Gain/1
  Sum1/1 -> Delay5/1
  Sum/1 -> Delay4/1
  Gain1/1 -> Sum/1
  Delay3/1 -> Sum/2
  Delay4/1 -> Sum1/2
  Gain3/1 -> Sum2/1
  Delay5/1 -> Sum2/2
  Gain/1 -> Delay3/1
  Sum2/1 -> Out1/1
  Gain2/1 -> Sum1/1

== system MIMO_FLOATING_POINT/Transceiver/Interpolation /E4 ==
  In1 : Inport
  Delay3 : Delay  DelayLength=1
  Delay4 : Delay  DelayLength=1
  Delay5 : Delay  DelayLength=1
  Gain : Gain
  Gain1 : Gain  Gain=161
  Gain2 : Gain  Gain=315
  Gain3 : Gain  Gain=35
  Sum : Sum
  Sum1 : Sum
  Sum2 : Sum
  Out1 : Outport
  wires:
  In1/1 -> Gain2/1, Gain3/1, Gain1/1, Gain/1
  Sum1/1 -> Delay5/1
  Sum/1 -> Delay4/1
  Gain1/1 -> Sum/1
  Delay3/1 -> Sum/2
  Delay4/1 -> Sum1/2
  Gain3/1 -> Sum2/1
  Delay5/1 -> Sum2/2
  Gain/1 -> Delay3/1
  Sum2/1 -> Out1/1
  Gain2/1 -> Sum1/1

== system MIMO_FLOATING_POINT/Transceiver/Interpolation /E5 ==
  In1 : Inport
  Delay6 : Delay  DelayLength=1
  Delay7 : Delay  DelayLength=1
  Gain4 : Gain  Gain=120
  Gain5 : Gain  Gain=336
  Gain6 : Gain  Gain=56
  Sum4 : Sum
  Sum5 : Sum
  Out1 : Outport
  wires:
  Gain4/1 -> Delay6/1
  In1/1 -> Gain6/1, Gain5/1, Gain4/1
  Sum5/1 -> Out1/1
  Sum4/1 -> Delay7/1
  Delay7/1 -> Sum5/2
  Gain6/1 -> Sum5/1
  Gain5/1 -> Sum4/1
  Delay6/1 -> Sum4/2

== system MIMO_FLOATING_POINT/Transceiver/Interpolation /E6 ==
  In1 : Inport
  Delay6 : Delay  DelayLength=1
  Delay7 : Delay  DelayLength=1
  Gain4 : Gain  Gain=84
  Gain5 : Gain  Gain=344
  Sum4 : Sum
  Sum5 : Sum
  Out1 : Outport
  wires:
  In1/1 -> Gain5/1, Gain4/1
  Sum5/1 -> Out1/1
  Sum4/1 -> Delay7/1
  Delay7/1 -> Sum5/2
  Gain4/1 -> Sum5/1, Delay6/1
  Gain5/1 -> Sum4/1
  Delay6/1 -> Sum4/2

== system MIMO_FLOATING_POINT/Transceiver/Interpolation /E7 ==
  In1 : Inport
  Delay6 : Delay  DelayLength=1
  Delay7 : Delay  DelayLength=1
  Gain4 : Gain  Gain=56
  Gain5 : Gain  Gain=336
  Gain6 : Gain  Gain=120
  Sum4 : Sum
  Sum5 : Sum
  Out1 : Outport
  wires:
  Gain4/1 -> Delay6/1
  In1/1 -> Gain6/1, Gain5/1, Gain4/1
  Sum5/1 -> Out1/1
  Sum4/1 -> Delay7/1
  Delay7/1 -> Sum5/2
  Gain6/1 -> Sum5/1
  Gain5/1 -> Sum4/1
  Delay6/1 -> Sum4/2

== system MIMO_FLOATING_POINT/Transceiver/Interpolation 1/E0 ==
  In1 : Inport
  Delay3 : Delay  DelayLength=1
  Delay4 : Delay  DelayLength=1
  Delay5 : Delay  DelayLength=1
  Gain : Gain  Gain=35
  Gain1 : Gain  Gain=315
  Gain2 : Gain  Gain=161
  Gain3 : Gain
  Sum : Sum
  Sum1 : Sum
  Sum2 : Sum
  Out1 : Outport
  wires:
  In1/1 -> Gain2/1, Gain3/1, Gain1/1, Gain/1
  Sum1/1 -> Delay5/1
  Sum/1 -> Delay4/1
  Gain1/1 -> Sum/1
  Delay3/1 -> Sum/2
  Delay4/1 -> Sum1/2
  Gain3/1 -> Sum2/1
  Delay5/1 -> Sum2/2
  Gain/1 -> Delay3/1
  Sum2/1 -> Out1/1
  Gain2/1 -> Sum1/1

== system MIMO_FLOATING_POINT/Transceiver/Interpolation 1/E0(Z) ==
  Input : Inport
  Delay : Delay  DelayLength=5
  Gain : Gain  Gain=0.5
  Out1 : Outport
  wires:
  Input/1 -> Gain/1
  Delay/1 -> Out1/1
  Gain/1 -> Delay/1

== system MIMO_FLOATING_POINT/Transceiver/Interpolation 1/E1 ==
  In1 : Inport
  Delay3 : Delay  DelayLength=1
  Delay4 : Delay  DelayLength=1
  Delay5 : Delay  DelayLength=1
  Gain : Gain  Gain=20
  Gain1 : Gain  Gain=284
  Gain2 : Gain  Gain=204
  Gain3 : Gain  Gain=4
  Sum : Sum
  Sum1 : Sum
  Sum2 : Sum
  Out1 : Outport
  wires:
  In1/1 -> Gain2/1, Gain3/1, Gain1/1, Gain/1
  Sum1/1 -> Delay5/1
  Sum/1 -> Delay4/1
  Gain1/1 -> Sum/1
  Delay3/1 -> Sum/2
  Delay4/1 -> Sum1/2
  Gain3/1 -> Sum2/1
  Delay5/1 -> Sum2/2
  Gain/1 -> Delay3/1
  Sum2/1 -> Out1/1
  Gain2/1 -> Sum1/1

== system MIMO_FLOATING_POINT/Transceiver/Interpolation 1/E1(Z) ==
  Input1 : Inport
  10-12 : Gain  Gain=0.3078
  2-20 : Gain  Gain=0.0011
  4-18 : Gain  Gain=-0.0072
  6-16 : Gain  Gain=0.0263
  8-14 : Gain  Gain=-0.078
  Add{7..10,12..16} (9 alike) : Sum
  Delay{21,23,25,27,29,31,33,35,37} (9 alike) : Delay  DelayLength=1
  Output : Outport
  wires:
  8-14/1 -> Add13/1, Add9/1
  Delay29/1 -> Add12/2  "x[n-11]"
  Add14/1 -> Delay35/1
  Input1/1 -> 2-20/1, 4-18/1, 6-16/1, 8-14/1, 10-12/1
  Add8/1 -> Delay25/1
  4-18/1 -> Add15/1, Add7/1
  Delay33/1 -> Add14/2  "x[n-15]"
  Add12/1 -> Delay31/1
  10-12/1 -> Add10/1, Add12/1
  Add9/1 -> Delay27/1
  Add16/1 -> Output/1
  Delay37/1 -> Add16/2  "x[n-19]"
  6-16/1 -> Add14/1, Add8/1
  Delay25/1 -> Add9/2  "x[n-7]"
  Add7/1 -> Delay23/1
  Add15/1 -> Delay37/1
  Delay23/1 -> Add8/2  "x[n-5]"
  Delay27/1 -> Add10/2  "x[n-9]"
  Delay31/1 -> Add13/2  "x[n-13]"
  Delay35/1 -> Add15/2  "x[n-17]"
  Delay21/1 -> Add7/2  "x[n-3]"
  2-20/1 -> Delay21/1, Add16/1
  Add13/1 -> Delay33/1
  Add10/1 -> Delay29/1

== system MIMO_FLOATING_POINT/Transceiver/Interpolation 1/E2 ==
  In1 : Inport
  Delay3 : Delay  DelayLength=1
  Delay4 : Delay  DelayLength=1
  Delay5 : Delay  DelayLength=1
  Gain : Gain  Gain=10
  Gain1 : Gain  Gain=246
  Sum : Sum
  Sum1 : Sum
  Sum2 : Sum
  Out1 : Outport
  wires:
  In1/1 -> Gain1/1, Gain/1
  Sum1/1 -> Delay5/1
  Sum/1 -> Delay4/1
  Gain1/1 -> Sum1/1, Sum/1
  Delay3/1 -> Sum/2
  Delay4/1 -> Sum1/2
  Gain/1 -> Sum2/1, Delay3/1
  Delay5/1 -> Sum2/2
  Sum2/1 -> Out1/1

== system MIMO_FLOATING_POINT/Transceiver/Interpolation 1/E3 ==
  In1 : Inport
  Delay3 : Delay  DelayLength=1
  Delay4 : Delay  DelayLength=1
  Delay5 : Delay  DelayLength=1
  Gain : Gain  Gain=4
  Gain1 : Gain  Gain=204
  Gain2 : Gain  Gain=284
  Gain3 : Gain  Gain=20
  Sum : Sum
  Sum1 : Sum
  Sum2 : Sum
  Out1 : Outport
  wires:
  In1/1 -> Gain2/1, Gain3/1, Gain1/1, Gain/1
  Sum1/1 -> Delay5/1
  Sum/1 -> Delay4/1
  Gain1/1 -> Sum/1
  Delay3/1 -> Sum/2
  Delay4/1 -> Sum1/2
  Gain3/1 -> Sum2/1
  Delay5/1 -> Sum2/2
  Gain/1 -> Delay3/1
  Sum2/1 -> Out1/1
  Gain2/1 -> Sum1/1

== system MIMO_FLOATING_POINT/Transceiver/Interpolation 1/E4 ==
  In1 : Inport
  Delay3 : Delay  DelayLength=1
  Delay4 : Delay  DelayLength=1
  Delay5 : Delay  DelayLength=1
  Gain : Gain
  Gain1 : Gain  Gain=161
  Gain2 : Gain  Gain=315
  Gain3 : Gain  Gain=35
  Sum : Sum
  Sum1 : Sum
  Sum2 : Sum
  Out1 : Outport
  wires:
  In1/1 -> Gain2/1, Gain3/1, Gain1/1, Gain/1
  Sum1/1 -> Delay5/1
  Sum/1 -> Delay4/1
  Gain1/1 -> Sum/1
  Delay3/1 -> Sum/2
  Delay4/1 -> Sum1/2
  Gain3/1 -> Sum2/1
  Delay5/1 -> Sum2/2
  Gain/1 -> Delay3/1
  Sum2/1 -> Out1/1
  Gain2/1 -> Sum1/1

== system MIMO_FLOATING_POINT/Transceiver/Interpolation 1/E5 ==
  In1 : Inport
  Delay6 : Delay  DelayLength=1
  Delay7 : Delay  DelayLength=1
  Gain4 : Gain  Gain=120
  Gain5 : Gain  Gain=336
  Gain6 : Gain  Gain=56
  Sum4 : Sum
  Sum5 : Sum
  Out1 : Outport
  wires:
  Gain4/1 -> Delay6/1
  In1/1 -> Gain6/1, Gain5/1, Gain4/1
  Sum5/1 -> Out1/1
  Sum4/1 -> Delay7/1
  Delay7/1 -> Sum5/2
  Gain6/1 -> Sum5/1
  Gain5/1 -> Sum4/1
  Delay6/1 -> Sum4/2

== system MIMO_FLOATING_POINT/Transceiver/Interpolation 1/E6 ==
  In1 : Inport
  Delay6 : Delay  DelayLength=1
  Delay7 : Delay  DelayLength=1
  Gain4 : Gain  Gain=84
  Gain5 : Gain  Gain=344
  Sum4 : Sum
  Sum5 : Sum
  Out1 : Outport
  wires:
  In1/1 -> Gain5/1, Gain4/1
  Sum5/1 -> Out1/1
  Sum4/1 -> Delay7/1
  Delay7/1 -> Sum5/2
  Gain4/1 -> Sum5/1, Delay6/1
  Gain5/1 -> Sum4/1
  Delay6/1 -> Sum4/2

== system MIMO_FLOATING_POINT/Transceiver/Interpolation 1/E7 ==
  In1 : Inport
  Delay6 : Delay  DelayLength=1
  Delay7 : Delay  DelayLength=1
  Gain4 : Gain  Gain=56
  Gain5 : Gain  Gain=336
  Gain6 : Gain  Gain=120
  Sum4 : Sum
  Sum5 : Sum
  Out1 : Outport
  wires:
  Gain4/1 -> Delay6/1
  In1/1 -> Gain6/1, Gain5/1, Gain4/1
  Sum5/1 -> Out1/1
  Sum4/1 -> Delay7/1
  Delay7/1 -> Sum5/2
  Gain6/1 -> Sum5/1
  Gain5/1 -> Sum4/1
  Delay6/1 -> Sum4/2

== system MIMO_FLOATING_POINT/Transceiver5/ADC 1/SigmaDelta ADC ==
  note: c1
  In : Inport
  Discrete Transfer Fcn : DiscreteTransferFcn  Denominator=[1 -1]
  Discrete Transfer Fcn1 : DiscreteTransferFcn  Numerator=[1 0]  Denominator=[1 -1]
  Discrete Transfer Fcn2 : DiscreteTransferFcn  Denominator=[1 -1]
  Discrete Transfer Fcn3 : DiscreteTransferFcn  Numerator=[1 0]  Denominator=[1 -1]
  Discrete Transfer Fcn4 : DiscreteTransferFcn  Denominator=[1 -1]
  Discrete Transfer Fcn5 : DiscreteTransferFcn  Numerator=[1 0]  Denominator=[1 -1]
  Sign : Signum
  Sum : Sum  Inputs=-++  InputSameDT=on  SaturateOnIntegerOverflow=on  OutDataTypeStr=Inherit: Same as first input
  Sum1 : Sum  Inputs=-+  InputSameDT=on  SaturateOnIntegerOverflow=on  OutDataTypeStr=Inherit: Same as first input
  Sum3 : Sum  Inputs=-+  InputSameDT=on  SaturateOnIntegerOverflow=on  OutDataTypeStr=Inherit: Same as first input
  Sum4 : Sum  Inputs=++++++  InputSameDT=on  SaturateOnIntegerOverflow=on  OutDataTypeStr=Inherit: Same as first input
  a : Gain  Gain=-1  SaturateOnIntegerOverflow=on  OutDataTypeStr=Inherit: Same as input  ParamDataTypeStr=Inherit: Same as input
  a1 : Gain  Gain=0.556869897897495  SaturateOnIntegerOverflow=on  OutDataTypeStr=Inherit: Same as input  ParamDataTypeStr=Inherit: Same as input
  a2 : Gain  Gain=-0.556869897925717  SaturateOnIntegerOverflow=on  OutDataTypeStr=Inherit: Same as input  ParamDataTypeStr=Inherit: Same as input
  a3 : Gain  Gain=5.57074843011795e-10  SaturateOnIntegerOverflow=on  OutDataTypeStr=Inherit: Same as input  ParamDataTypeStr=Inherit: Same as input
  a4 : Gain  Gain=-0.239860502762260  SaturateOnIntegerOverflow=on  OutDataTypeStr=Inherit: Same as input  ParamDataTypeStr=Inherit: Same as input
  a5 : Gain  Gain=-0.0411685762497780  SaturateOnIntegerOverflow=on  OutDataTypeStr=Inherit: Same as input  ParamDataTypeStr=Inherit: Same as input
  a6 : Gain  Gain=0.0229325751731016  SaturateOnIntegerOverflow=on  OutDataTypeStr=Inherit: Same as input  ParamDataTypeStr=Inherit: Same as input
  gc1 : Gain  Gain=2.00000000000000  SaturateOnIntegerOverflow=on  OutDataTypeStr=Inherit: Same as input  ParamDataTypeStr=Inherit: Same as input
  gc2 : Gain  Gain=2.07602752770857  SaturateOnIntegerOverflow=on  OutDataTypeStr=Inherit: Same as input  ParamDataTypeStr=Inherit: Same as input
  gc3 : Gain  Gain=1.92397247229143  SaturateOnIntegerOverflow=on  OutDataTypeStr=Inherit: Same as input  ParamDataTypeStr=Inherit: Same as input
  Out : Outport
  wires:
  gc1/1 -> Sum/1
  a5/1 -> Sum4/2
  Discrete Transfer Fcn2/1 -> Discrete Transfer Fcn3/1, a3/1
  Sum4/1 -> Sign/1
  Sum1/1 -> Discrete Transfer Fcn2/1
  Sum/1 -> Discrete Transfer Fcn/1
  a1/1 -> Sum4/6
  gc2/1 -> Sum1/1
  a/1 -> Sum/3
  Discrete Transfer Fcn3/1 -> a4/1, Sum3/2, gc2/1
  Discrete Transfer Fcn5/1 -> a6/1, gc3/1
  Discrete Transfer Fcn1/1 -> a2/1, gc1/1, Sum1/2
  In/1 -> Sum/2
  Sign/1 -> Out/1, a/1
  gc3/1 -> Sum3/1
  a3/1 -> Sum4/4
  a4/1 -> Sum4/3
  a2/1 -> Sum4/5
  Discrete Transfer Fcn/1 -> Discrete Transfer Fcn1/1, a1/1
  Sum3/1 -> Discrete Transfer Fcn4/1
  Discrete Transfer Fcn4/1 -> Discrete Transfer Fcn5/1, a5/1
  a6/1 -> Sum4/1

== system MIMO_FLOATING_POINT/Transceiver5/Interpolation /E0 ==
  In1 : Inport
  Delay3 : Delay  DelayLength=1
  Delay4 : Delay  DelayLength=1
  Delay5 : Delay  DelayLength=1
  Gain : Gain  Gain=35
  Gain1 : Gain  Gain=315
  Gain2 : Gain  Gain=161
  Gain3 : Gain
  Sum : Sum
  Sum1 : Sum
  Sum2 : Sum
  Out1 : Outport
  wires:
  In1/1 -> Gain2/1, Gain3/1, Gain1/1, Gain/1
  Sum1/1 -> Delay5/1
  Sum/1 -> Delay4/1
  Gain1/1 -> Sum/1
  Delay3/1 -> Sum/2
  Delay4/1 -> Sum1/2
  Gain3/1 -> Sum2/1
  Delay5/1 -> Sum2/2
  Gain/1 -> Delay3/1
  Sum2/1 -> Out1/1
  Gain2/1 -> Sum1/1

== system MIMO_FLOATING_POINT/Transceiver5/Interpolation /E0(Z) ==
  Input : Inport
  Delay : Delay  DelayLength=5
  Gain : Gain  Gain=0.5
  Out1 : Outport
  wires:
  Input/1 -> Gain/1
  Delay/1 -> Out1/1
  Gain/1 -> Delay/1

== system MIMO_FLOATING_POINT/Transceiver5/Interpolation /E1 ==
  In1 : Inport
  Delay3 : Delay  DelayLength=1
  Delay4 : Delay  DelayLength=1
  Delay5 : Delay  DelayLength=1
  Gain : Gain  Gain=20
  Gain1 : Gain  Gain=284
  Gain2 : Gain  Gain=204
  Gain3 : Gain  Gain=4
  Sum : Sum
  Sum1 : Sum
  Sum2 : Sum
  Out1 : Outport
  wires:
  In1/1 -> Gain2/1, Gain3/1, Gain1/1, Gain/1
  Sum1/1 -> Delay5/1
  Sum/1 -> Delay4/1
  Gain1/1 -> Sum/1
  Delay3/1 -> Sum/2
  Delay4/1 -> Sum1/2
  Gain3/1 -> Sum2/1
  Delay5/1 -> Sum2/2
  Gain/1 -> Delay3/1
  Sum2/1 -> Out1/1
  Gain2/1 -> Sum1/1
